simulink model "EKFguidanceloop"  (R2019b)
settings: Solver=VariableStepAuto  StartTime=0.0  StopTime=9.99  RelTol=1e-3
settings Model: Creator=win10  LastModifiedBy=win10

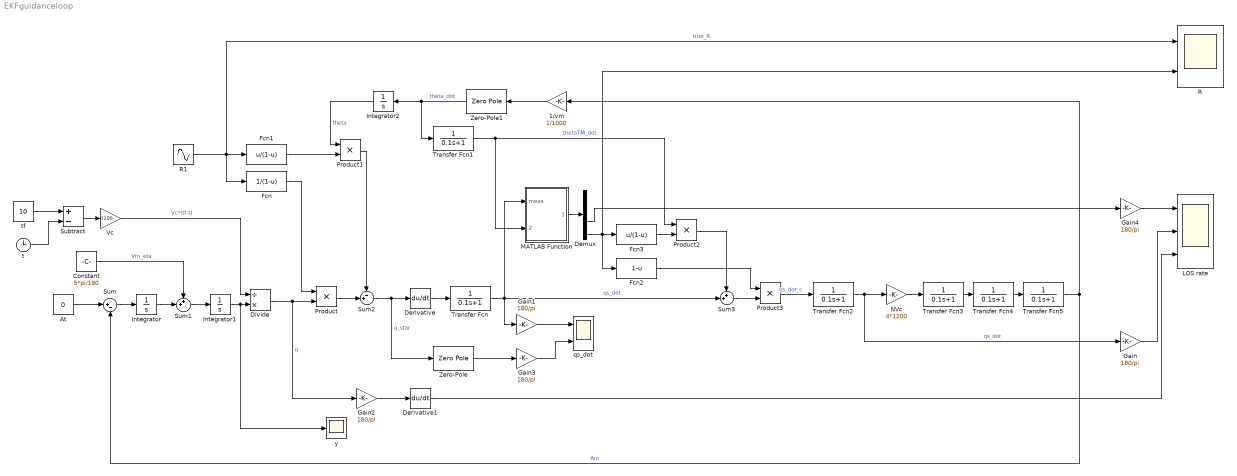
== system EKFguidanceloop ==
  1/vm : Gain  Gain=1/1000
  At : Constant  Value=0
  Constant : Constant  Value=5*pi/180
  Demux : Demux
  Derivative : Derivative
  Derivative1 : Derivative
  Divide : Product  Inputs=/*
  Fcn : Fcn  Expr=1/(1-u)
  Fcn1 : Fcn  Expr=u/(1-u)
  Fcn2 : Fcn  Expr=1-u
  Fcn3 : Fcn  Expr=u/(1-u)
  Gain{,1..4} (5 alike) : Gain  Gain=180/pi
  Integrator : Integrator
  Integrator1 : Integrator
  Integrator2 : Integrator
  LOS rate : Scope  NumInputPorts=3
  MATLAB Function : MATLAB Function  TreatAsAtomicUnit=on
  NVc : Gain  Gain=4*1200
  Product{,1..3} (4 alike) : Product
  R : Scope  NumInputPorts=2
  R1 : Sin  Amplitude=0.06  Frequency=pi/2  SampleTime=0
  Subtract : Sum  Inputs=+-
  Sum : Sum  Inputs=|+-
  Sum1 : Sum  Inputs=++|
  Sum2 : Sum  Inputs=-+|
  Sum3 : Sum  Inputs=++|
  Transfer Fcn{,1..5} (6 alike) : TransferFcn  Denominator=[0.1 1]
  Vc : Gain  Gain=1200
  Zero-Pole : ZeroPole  Zeros=[0]  Poles=[-10]  Gain=[10]
  Zero-Pole1 : ZeroPole  Zeros=[-0.5]  Poles=[-100000]  Gain=[200000]
  qs_dot : Scope  NumInputPorts=2
  t : Clock
  tf : Constant  Value=10
  y : Scope
  wires:
  At/1 -> Sum/1
  Sum/1 -> Integrator/1
  Constant/1 -> Sum1/1  "Vm_eta"
  t/1 -> Subtract/2
  tf/1 -> Subtract/1
  Subtract/1 -> Vc/1
  Vc/1 -> Divide/1  "Vc*(tf-t)"
  Integrator1/1 -> y/1, Divide/2
  R1/1 -> R/1, Fcn/1, Fcn1/1  "true_R"
  Divide/1 -> Gain2/1, Product/2  "q"
  Fcn/1 -> Product/1
  Derivative/1 -> Transfer Fcn/1
  Product/1 -> Sum2/2
  Gain2/1 -> Derivative1/1
  Derivative1/1 -> LOS rate/3
  Sum2/1 -> Zero-Pole/1, Derivative/1  "q_star"
  Zero-Pole/1 -> Gain3/1
  Transfer Fcn/1 -> MATLAB Function/1(meas), Sum3/2, Gain1/1  "qs_dot"
  Product1/1 -> Sum2/1
  Gain1/1 -> qs_dot/1
  Gain3/1 -> qs_dot/2
  Fcn1/1 -> Product1/2
  Integrator2/1 -> Product1/1  "theta"
  Zero-Pole1/1 -> Transfer Fcn1/1, Integrator2/1  "theta_dot"
  Transfer Fcn1/1 -> MATLAB Function/2(thetaTM_dot), Product2/1  "thetaTM_dot"
  MATLAB Function/1(xhatOut) -> Demux/1
  Demux/4 -> R/2, Fcn2/1, Fcn3/1
  1/vm/1 -> Zero-Pole1/1
  Fcn3/1 -> Product2/2
  Product2/1 -> Sum3/1
  Sum3/1 -> Product3/2
  Fcn2/1 -> Product3/1
  Product3/1 -> Transfer Fcn2/1  "qs_dot_c"
  Transfer Fcn2/1 -> Gain/1, NVc/1  "qs_dot"
  NVc/1 -> Transfer Fcn3/1
  Transfer Fcn3/1 -> Transfer Fcn4/1
  Transfer Fcn4/1 -> Transfer Fcn5/1
  Transfer Fcn5/1 -> 1/vm/1, Sum/2  "Am"
  Demux/3 -> Gain4/1
  Sum1/1 -> Integrator1/1
  Integrator/1 -> Sum1/2
  Gain4/1 -> LOS rate/1
  Gain/1 -> LOS rate/2

== matlab function EKFguidanceloop/MATLAB Function ==
  settings: updateMethod=DISCRETE  sampleTime=0.1
  data: meas input; xhatOut output; thetaTM_dot input
function xhatOut = ExtKalman_Simulink(meas,thetaTM_dot)
% This Embedded MATLAB Function implements an extended Kalman filter used
% for target tracking.
%
% The continuous-time process model is given by
% dx/dt = A*x + B*w

% where, x = [q q_dot qst_dot rou]', q,q_dot is true LOS angle and LOS rate 
% qst_dot is true output of LOS rate from seeker, rou is the radome error
% slope. w = [0 w2 0  w4]'

% Discretize the LTI system model.
%x_k+1 = D*x_k + E*w_k

% and the measurements are given by
% y = qst_dot/(1-rou) - rou/(1-rou)*thetaTM_dot

% Define storage for the variables that need to persist
% between time periods.
Td = 0.1;
dt = 0.1;

persistent P xhat Q R
if isempty(P)
% First time through the code so do some initialization
 xhat = [0;0;0;0];
 P = diag([10 10 10 1]);
 Q = diag([0 1e-5/dt 0 1e-3/dt]);
 R = diag([0.04*pi*pi/180/180]);
end


% Calculate the Jacobians for the state equations
% Dynamic state transition matrix in continous-time domain.
A = [0 1 0 0;
     0 0 0 0;
     0 1/Td -1/Td 0;
     0 0 0 0];
  
% noise matrix in continous-time domain.
B = eye(4);
 
% system matrix in discrete-time domain.
% D = expm(A*dt); 
% E = B*dt;

D = [1 dt 0 0;
     0 1 0 0;
     0 dt/Td 1-dt/Td 0;
     0 0 0 1];
E = [dt 0 0 0;
      0 dt 0 0;
      0 0 dt 0;
      0 0 0 dt];
  
% Calculate the Jacobians for the measurement equations
   q = xhat(1);
   q_dot = xhat(2);
   qst_dot = xhat(3);  
   rou = xhat(4);
   
yhat = qst_dot/(1-rou) - rou/(1-rou)*thetaTM_dot;

H = [0 0 1/(1-rou) (qst_dot-thetaTM_dot)/(1-rou)^2];
  
% Propogate the state and covariance matrices
xhat = D*xhat;
% xhat = xhat + A*xhat*dt;
P = D*P*D' + E*Q*E';
  
% Calculate the Kalman gain
K = P*H'/(H*P*H' + R);
% Calculate the measurement residual
resid = meas - yhat;
% Update the state and covariance estimates
xhat = xhat + K*resid;
P = (eye(size(K,1))-K*H)*P;
% Post the results
xhatOut = xhat;


% rangeHat = sqrt(xhat(1)^2+xhat(3)^2);
% bearingHat = atan2(xhat(3),xhat(1));
% yu = [thetaM;psiM];
% yhat = MeasurementModel(xhat);
% H = [cos(bearingHat) 0 sin(bearingHat) 0;
%  -sin(bearingHat)/rangeHat 0 cos(bearingHat)/rangeHat 0];
% % Propogate the state and covariance matrices
% xhat = F*xhat;
% P = F*P*F' + Q;
% % Calculate the Kalman gain
% K = P*H'/(H*P*H' + R);
% % Calculate the measurement residual
% resid = meas - yhat;
% % Update the state and covariance estimates
% xhat = xhat + K*resid;
% P = (eye(size(K,1))-K*H)*P;
% % Post the results
% xhatOut = xhat;
% y = u;
